simulink model "PPM"  (R2020b)
settings: Solver=VariableStepAuto  StartTime=0.0  StopTime=10.0  RelTol=1e-3
libraries: powerlib_meascontrol x2, simulink x1
settings Model: Creator=MEDIA  LastModifiedBy=MEDIA

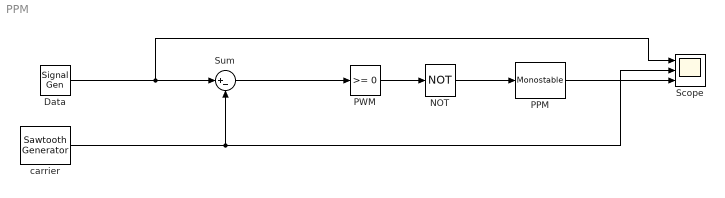
== system PPM ==
  Data : SignalGenerator  Amplitude=0.9  Units=rad/sec
  NOT : Logic  Operator=NOT  IconShape=distinctive  AllPortsSameDT=off  OutDataTypeStr=boolean
  PPM : powerlib_meascontrol/Logic/Monostable  EdgeDetect=Rising  PulseDuration=0.015  ic=0  Ts=0
      settings: SourceProductBaseCode=PS
  PWM : simulink/Logic and Bit Operations/Compare To Zero  relop=>=  OutDataTypeStr=boolean  ZeroCross=off
  Scope : Scope  NumInputPorts=3
  Sum : Sum  Inputs=|+-
  carrier : powerlib_meascontrol/Pulse & Signal Generators/Sawtooth Generator  Freq=1  Phase=0  Ts=0
  wires:
  carrier/1 -> Scope/2, Sum/2
  Sum/1 -> PWM/1
  Data/1 -> Scope/1, Sum/1
  PWM/1 -> NOT/1
  NOT/1 -> PPM/1
  PPM/1 -> Scope/3
